simulink model "stereo_ibvs_core_backup_20260724_010158"  (R2025b)
settings: Solver=FixedStepDiscrete  StartTime=0.0  StopTime=10  FixedStep=cfg.Ts  RelTol=1e-3
InitFcn:
  | modelPath = get_param(bdroot,'FileName');
  |                                                                                       simulinkPath = fileparts(fileparts(modelPath));
  |                                                                                       configPath = fullfile(simulinkPath,'config','stereo_ibvs_config.m');
  |                                                                                       if ~isfile(configPath), error('StereoIBVS:ConfigNotFound','找不到配置文件：%s',configPath); end
  |                                                                                       run(configPath);
undefined symbols (not defined in the file): cfg
(part 3 of 4)

== matlab function stereo_ibvs_core_backup_20260724_010158/08_Zoom_Controller/08A Right Visibility Guard/Right Visibility Guard ==
  data: xLeftMeasured input; uRightPredicted output; rhoHatSafe input; focalLengthMeasuredMm input; focalLengthDataValid input; cameraModelValid input; validLeft input; validRight input; ekfPredictionValid input; rightReacquireActive input; resetSafe input; scaleDesired input; numericalEpsilon input; baseline input; outputPixelPitchXmm input; cxR input; focalLengthHardwareMaxMm input; visibilityEpsilon input; imageWidthPx input; rightVisibilityMarginPx input; focalLengthWorkingMaxMm input; focalLengthWorkingMinMm input; targetCharacteristicSize input; rightVisibilityHysteresisPx input; rightVisibilityMarginActualPx output; fRightMaxVisibleMm output; fRightMaxEffectiveMm output; rightScaleDesiredEffective output; rightVisibilityActive output; rightVisibilityInfeasible output; scaleDesiredEffective output; rightScaleDesiredNominal output; fRightMeasuredMm output
function [ ...
    uRightPredicted, ...
    rightVisibilityMarginActualPx, ...
    fRightMaxVisibleMm, ...
    fRightMaxEffectiveMm, ...
    rightScaleDesiredEffective, ...
    rightVisibilityActive, ...
    rightVisibilityInfeasible, ...
    scaleDesiredEffective, ...
    rightScaleDesiredNominal, ...
    fRightMeasuredMm] = fcn( ...
    xLeftMeasured, ...
    rhoHatSafe, ...
    focalLengthMeasuredMm, ...
    focalLengthDataValid, ...
    cameraModelValid, ...
    validLeft, ...
    validRight, ...
    ekfPredictionValid, ...
    rightReacquireActive, ...
    resetSafe, ...
    scaleDesired, ...
    numericalEpsilon, ...
    baseline, ...
    outputPixelPitchXmm, ...
    cxR, ...
    focalLengthHardwareMaxMm, ...
    visibilityEpsilon, ...
    imageWidthPx, ...
    rightVisibilityMarginPx, ...
    focalLengthWorkingMaxMm, ...
    focalLengthWorkingMinMm, ...
    targetCharacteristicSize, ...
    rightVisibilityHysteresisPx)
%#codegen
% 右相机可见性保护。
% 所有配置参数均由外部 Constant 块输入。

persistent active

if isempty(active)
    active = 1;
end

if resetSafe > 0.5
    active = 1;
end

%% 默认安全输出
uRightPredicted = cxR;
rightVisibilityMarginActualPx = 0;

fRightMaxVisibleMm = 0;
fRightMaxEffectiveMm = ...
    focalLengthWorkingMinMm(2);

rightScaleDesiredNominal = ...
    scaleDesired(2);

rightScaleDesiredEffective = ...
    rightScaleDesiredNominal;

scaleDesiredEffective = ...
    scaleDesired;

rightVisibilityActive = 1;
rightVisibilityInfeasible = 1;

fRightMeasuredMm = 0;

%% 输入检查
inputFinite = ...
    isfinite(xLeftMeasured) && ...
    isfinite(rhoHatSafe) && ...
    all(isfinite(focalLengthMeasuredMm)) && ...
    all(isfinite(scaleDesired)) && ...
    isfinite(numericalEpsilon) && ...
    isfinite(baseline) && ...
    isfinite(outputPixelPitchXmm) && ...
    isfinite(cxR) && ...
    all(isfinite(focalLengthHardwareMaxMm)) && ...
    isfinite(visibilityEpsilon) && ...
    isfinite(imageWidthPx) && ...
    isfinite(rightVisibilityMarginPx) && ...
    all(isfinite(focalLengthWorkingMaxMm)) && ...
    all(isfinite(focalLengthWorkingMinMm)) && ...
    isfinite(targetCharacteristicSize) && ...
    isfinite(rightVisibilityHysteresisPx);

modelReady = ...
    focalLengthDataValid > 0.5 && ...
    cameraModelValid > 0.5 && ...
    outputPixelPitchXmm > numericalEpsilon;

if ~inputFinite || ~modelReady
    active = 1;
    return;
end

%% 右相机预测位置
fRightMeasuredMm = ...
    focalLengthMeasuredMm(2);

rho = max( ...
    rhoHatSafe, ...
    numericalEpsilon);

xRightPredicted = ...
    xLeftMeasured - ...
    baseline * rho;

fRightPx = ...
    focalLengthMeasuredMm(2) / ...
    outputPixelPitchXmm;

uRightPredicted = ...
    cxR + ...
    fRightPx * xRightPredicted;

rightVisibilityMarginActualPx = min( ...
    uRightPredicted, ...
    imageWidthPx - uRightPredicted);

%% 可见焦距上限
hardwareMaxPx = ...
    focalLengthHardwareMaxMm(2) / ...
    outputPixelPitchXmm;

if xRightPredicted < -visibilityEpsilon

    fMaxPx = ...
        (cxR - rightVisibilityMarginPx) / ...
        (-xRightPredicted);

elseif xRightPredicted > visibilityEpsilon

    fMaxPx = ...
        (imageWidthPx - ...
        rightVisibilityMarginPx - ...
        cxR) / ...
        xRightPredicted;

else
    fMaxPx = hardwareMaxPx;
end

fMaxPx = max(fMaxPx, 0);

fRightMaxVisibleMm = ...
    fMaxPx * outputPixelPitchXmm;

rawEffectiveMaxMm = min([
    focalLengthWorkingMaxMm(2)
    focalLengthHardwareMaxMm(2)
    fRightMaxVisibleMm
]);

rightVisibilityInfeasible = double( ...
    rawEffectiveMaxMm < ...
    focalLengthWorkingMinMm(2));

fRightMaxEffectiveMm = max( ...
    focalLengthWorkingMinMm(2), ...
    rawEffectiveMaxMm);

%% 调整右相机期望尺度
scaleRightMaxVisible = ...
    targetCharacteristicSize * ...
    fMaxPx * rho;

rightScaleDesiredEffective = min( ...
    rightScaleDesiredNominal, ...
    max(scaleRightMaxVisible, numericalEpsilon));

scaleDesiredEffective = [
    scaleDesired(1)
    rightScaleDesiredEffective
];

%% 滞回状态
enterGuard = ...
    validLeft <= 0.5 || ...
    validRight <= 0.5 || ...
    ekfPredictionValid <= 0.5 || ...
    rightReacquireActive > 0.5 || ...
    rightVisibilityInfeasible > 0.5 || ...
    uRightPredicted < rightVisibilityMarginPx || ...
    uRightPredicted > ...
        imageWidthPx - rightVisibilityMarginPx || ...
    focalLengthMeasuredMm(2) > ...
        fRightMaxEffectiveMm + numericalEpsilon;

exitGuard = ...
    validLeft > 0.5 && ...
    validRight > 0.5 && ...
    ekfPredictionValid > 0.5 && ...
    rightReacquireActive <= 0.5 && ...
    rightVisibilityInfeasible <= 0.5 && ...
    uRightPredicted >= ...
        rightVisibilityMarginPx + ...
        rightVisibilityHysteresisPx && ...
    uRightPredicted <= ...
        imageWidthPx - ...
        rightVisibilityMarginPx - ...
        rightVisibilityHysteresisPx && ...
    focalLengthMeasuredMm(2) <= ...
        fRightMaxEffectiveMm;

if enterGuard
    active = 1;
elseif exitGuard
    active = 0;
end

rightVisibilityActive = ...
    double(active > 0.5);

%% 输出保护
if any(~isfinite([
        uRightPredicted
        rightVisibilityMarginActualPx
        fRightMaxVisibleMm
        fRightMaxEffectiveMm
        rightScaleDesiredEffective
        scaleDesiredEffective
        fRightMeasuredMm]))

    active = 1;

    uRightPredicted = cxR;
    rightVisibilityMarginActualPx = 0;

    fRightMaxVisibleMm = 0;
    fRightMaxEffectiveMm = ...
        focalLengthWorkingMinMm(2);

    rightScaleDesiredEffective = ...
        numericalEpsilon;

    scaleDesiredEffective = [
        scaleDesired(1)
        rightScaleDesiredEffective
    ];

    rightVisibilityActive = 1;
    rightVisibilityInfeasible = 1;
    fRightMeasuredMm = 0;
end
end

== matlab function stereo_ibvs_core_backup_20260724_010158/08_Zoom_Controller/08B_Zoom_Controller_Mm/V2 Zoom Controller ==
  data: focalLengthMeasuredMm input; fDotMmCmd output; focalLengthFresh input; focalLengthDataValid input; cameraModelValid input; scaleMeasured input; rhoHatSafe input; rhoDotHat input; scaleDesiredEffective input; validLeft input; ekfPredictionValid input; focalAtWorkingLowerLimit input; focalAtWorkingUpperLimit input; fRightMaxEffectiveMm input; rightVisibilityActive input; rightReacquireActive input; numericalEpsilon input; focalLengthWorkingMaxMm input; robustEnable input; betaF input; epsilonF input; Kf input; targetCharacteristicSize input; outputPixelPitchXmm input; focalLengthWorkingMinMm input; rightReacquireZoomRateMmPerSec input; focalRateDesignMmPerSec input; Ts input; focalRateGuaranteedMmPerSec input; focalRateAbsoluteMaxMmPerSec input; zoomControlEnable input; fDotMmLimited output; scaleError output; gDotCmd output; focalCommandOutwardAtWorkingLimit output; focalFeasible output; focalRateUsageGuaranteedCmd output; focalRateUsageHardCmd output
function [ ...
    fDotMmCmd, ...
    fDotMmLimited, ...
    scaleError, ...
    gDotCmd, ...
    focalCommandOutwardAtWorkingLimit, ...
    focalFeasible, ...
    focalRateUsageGuaranteedCmd, ...
    focalRateUsageHardCmd] = fcn( ...
    focalLengthMeasuredMm, ...
    focalLengthFresh, ...
    focalLengthDataValid, ...
    cameraModelValid, ...
    scaleMeasured, ...
    rhoHatSafe, ...
    rhoDotHat, ...
    scaleDesiredEffective, ...
    validLeft, ...
    ekfPredictionValid, ...
    focalAtWorkingLowerLimit, ...
    focalAtWorkingUpperLimit, ...
    fRightMaxEffectiveMm, ...
    rightVisibilityActive, ...
    rightReacquireActive, ...
    numericalEpsilon, ...
    focalLengthWorkingMaxMm, ...
    robustEnable, ...
    betaF, ...
    epsilonF, ...
    Kf, ...
    targetCharacteristicSize, ...
    outputPixelPitchXmm, ...
    focalLengthWorkingMinMm, ...
    rightReacquireZoomRateMmPerSec, ...
    focalRateDesignMmPerSec, ...
    Ts, ...
    focalRateGuaranteedMmPerSec, ...
    focalRateAbsoluteMaxMmPerSec, ...
    zoomControlEnable)
%#codegen
% V2 Zoom控制器。
% 焦距单位mm，速度命令单位mm/s。
% 所有配置参数均由外部 Constant 块输入。

%% 固定尺寸输出
fDotMmCmd = zeros(2,1);
fDotMmLimited = zeros(2,1);

scaleError = zeros(2,1);
gDotCmd = zeros(2,1);

focalCommandOutwardAtWorkingLimit = ...
    zeros(2,1);

focalFeasible = zeros(2,1);

focalRateUsageGuaranteedCmd = ...
    zeros(2,1);

focalRateUsageHardCmd = ...
    zeros(2,1);

%% 输入检查
inputFinite = ...
    all(isfinite(focalLengthMeasuredMm)) && ...
    all(isfinite(scaleMeasured)) && ...
    isfinite(rhoHatSafe) && ...
    all(isfinite(rhoDotHat)) && ...
    all(isfinite(scaleDesiredEffective)) && ...
    all(isfinite(focalAtWorkingLowerLimit)) && ...
    all(isfinite(focalAtWorkingUpperLimit)) && ...
    isfinite(fRightMaxEffectiveMm) && ...
    isfinite(numericalEpsilon) && ...
    all(isfinite(focalLengthWorkingMaxMm)) && ...
    isfinite(robustEnable) && ...
    all(isfinite(betaF)) && ...
    all(isfinite(epsilonF)) && ...
    all(isfinite(Kf(:))) && ...
    isfinite(targetCharacteristicSize) && ...
    isfinite(outputPixelPitchXmm) && ...
    all(isfinite(focalLengthWorkingMinMm)) && ...
    isfinite(rightReacquireZoomRateMmPerSec) && ...
    isfinite(focalRateDesignMmPerSec) && ...
    isfinite(Ts) && ...
    isfinite(focalRateGuaranteedMmPerSec) && ...
    isfinite(focalRateAbsoluteMaxMmPerSec) && ...
    isfinite(zoomControlEnable);

if ~inputFinite || ...
        numericalEpsilon <= 0 || ...
        outputPixelPitchXmm <= numericalEpsilon || ...
        Ts <= 0

    return;
end

rho = max(rhoHatSafe, numericalEpsilon);

upperEffectiveMm = [
    focalLengthWorkingMaxMm(1)
    fRightMaxEffectiveMm
];

%% V2控制律
for cameraIndex = 1:2

    scaleCurrent = max( ...
        scaleMeasured(cameraIndex), ...
        numericalEpsilon);

    scaleDesiredCurrent = max( ...
        scaleDesiredEffective(cameraIndex), ...
        numericalEpsilon);

    scaleError(cameraIndex) = ...
        log(scaleCurrent / scaleDesiredCurrent);

    depthRateEstimate = ...
        rhoDotHat(cameraIndex) / rho;

    robustTerm = 0;

    if robustEnable > 0.5
        robustTerm = ...
            betaF(cameraIndex) * ...
            scaleError(cameraIndex) / ...
            (abs(scaleError(cameraIndex)) + ...
            epsilonF(cameraIndex));
    end

    gDotCmd(cameraIndex) = ...
        -Kf(cameraIndex,cameraIndex) * ...
        scaleError(cameraIndex) - ...
        depthRateEstimate - ...
        robustTerm;

    fDotMmCmd(cameraIndex) = ...
        focalLengthMeasuredMm(cameraIndex) * ...
        gDotCmd(cameraIndex);

    focalRequiredMm = ...
        scaleDesiredEffective(cameraIndex) / ...
        (targetCharacteristicSize * rho) * ...
        outputPixelPitchXmm;

    focalFeasible(cameraIndex) = double( ...
        focalRequiredMm >= ...
            focalLengthWorkingMinMm(cameraIndex) && ...
        focalRequiredMm <= ...
            upperEffectiveMm(cameraIndex));
end

%% 焦距反馈超时或模型失效：Zoom立即停止
zoomInputValid = ...
    focalLengthFresh > 0.5 && ...
    focalLengthDataValid > 0.5 && ...
    cameraModelValid > 0.5;

if ~zoomInputValid || ...
        zoomControlEnable <= 0.5

    fDotMmCmd = zeros(2,1);
    fDotMmLimited = zeros(2,1);
    gDotCmd = zeros(2,1);
    return;
end

%% 右相机可见性保护
if rightVisibilityActive > 0.5 || ...
        rightReacquireActive > 0.5

    if focalLengthMeasuredMm(2) > ...
            fRightMaxEffectiveMm + numericalEpsilon

        fDotMmCmd(2) = ...
            -rightReacquireZoomRateMmPerSec;
    else
        fDotMmCmd(2) = ...
            min(fDotMmCmd(2), 0);
    end
end

%% 左相机或EKF无效：保留V2安全缩焦
if validLeft <= 0.5 || ...
        ekfPredictionValid <= 0.5

    fDotMmCmd = zeros(2,1);

    for cameraIndex = 1:2
        if focalLengthMeasuredMm(cameraIndex) > ...
                focalLengthWorkingMinMm(cameraIndex)

            fDotMmCmd(cameraIndex) = ...
                -rightReacquireZoomRateMmPerSec;
        end
    end
end

%% 工作范围方向诊断
for cameraIndex = 1:2

    focalCommandOutwardAtWorkingLimit(cameraIndex) = ...
        double( ...
        (focalAtWorkingLowerLimit(cameraIndex) > 0.5 && ...
        fDotMmCmd(cameraIndex) < 0) || ...
        (focalAtWorkingUpperLimit(cameraIndex) > 0.5 && ...
        fDotMmCmd(cameraIndex) > 0) || ...
        (focalLengthMeasuredMm(cameraIndex) >= ...
        upperEffectiveMm(cameraIndex) && ...
        fDotMmCmd(cameraIndex) > 0));
end

%% V2设计速度限制
fDotMmLimited = min( ...
    max( ...
        fDotMmCmd, ...
        -focalRateDesignMmPerSec), ...
    focalRateDesignMmPerSec);

%% 防止下一周期越过右相机可见焦距上限
nextRightFocalLengthMm = ...
    focalLengthMeasuredMm(2) + ...
    Ts * fDotMmLimited(2);

if focalLengthMeasuredMm(2) <= ...
        fRightMaxEffectiveMm && ...
        nextRightFocalLengthMm > ...
        fRightMaxEffectiveMm

    fDotMmLimited(2) = min( ...
        fDotMmLimited(2), ...
        (fRightMaxEffectiveMm - ...
        focalLengthMeasuredMm(2)) / Ts);
end

%% 速度使用率
if focalRateGuaranteedMmPerSec > numericalEpsilon
    focalRateUsageGuaranteedCmd = ...
        abs(fDotMmLimited) / ...
        focalRateGuaranteedMmPerSec;
end

if focalRateAbsoluteMaxMmPerSec > numericalEpsilon
    focalRateUsageHardCmd = ...
        abs(fDotMmLimited) / ...
        focalRateAbsoluteMaxMmPerSec;
end

%% 输出有限值保护
if any(~isfinite(fDotMmCmd)) || ...
        any(~isfinite(fDotMmLimited)) || ...
        any(~isfinite(scaleError)) || ...
        any(~isfinite(gDotCmd)) || ...
        any(~isfinite(focalFeasible)) || ...
        any(~isfinite(focalRateUsageGuaranteedCmd)) || ...
        any(~isfinite(focalRateUsageHardCmd))

    fDotMmCmd = zeros(2,1);
    fDotMmLimited = zeros(2,1);

    scaleError = zeros(2,1);
    gDotCmd = zeros(2,1);

    focalCommandOutwardAtWorkingLimit = ...
        zeros(2,1);

    focalFeasible = zeros(2,1);

    focalRateUsageGuaranteedCmd = ...
        zeros(2,1);

    focalRateUsageHardCmd = ...
        zeros(2,1);
end
end

== matlab function stereo_ibvs_core_backup_20260724_010158/08_Zoom_Controller/08C_Zoom_Priority_Supervisor/V2 Zoom Priority Supervisor ==
  data: scaleError input; depthTaskWeight output; depthErrorDelayed input; focalLengthMeasuredMm input; focalLengthFresh input; focalLengthDataValid input; cameraModelValid input; focalAtWorkingLowerLimit input; focalAtWorkingUpperLimit input; focalHeadroomMm input; focalFeasible input; validLeft input; validStereoQualified input; ekfPredictionValid input; resetSafe input; focalCommandOutwardAtWorkingLimit input; focalRateUsageGuaranteedCmd input; focalRateUsageHardCmd input; rightReacquireActive input; Ts input; zoomPriorityEnable input; armDepthRampTime input; scaleErrorEnterThreshold input; scaleErrorExitThreshold input; scaleSettledHoldTime input; disturbanceConfirmTime input; zoomOnlyMaxTime input; schedulerMode output; zoomPriorityActive output; zoomPriorityTimer output; scaleSettledTimer output; armRecoveryReason output; newDisturbanceDetected output
function [ ...
    depthTaskWeight, ...
    schedulerMode, ...
    zoomPriorityActive, ...
    zoomPriorityTimer, ...
    scaleSettledTimer, ...
    armRecoveryReason, ...
    newDisturbanceDetected] = fcn( ...
    scaleError, ...
    depthErrorDelayed, ...
    focalLengthMeasuredMm, ...
    focalLengthFresh, ...
    focalLengthDataValid, ...
    cameraModelValid, ...
    focalAtWorkingLowerLimit, ...
    focalAtWorkingUpperLimit, ...
    focalHeadroomMm, ...
    focalFeasible, ...
    validLeft, ...
    validStereoQualified, ...
    ekfPredictionValid, ...
    resetSafe, ...
    focalCommandOutwardAtWorkingLimit, ...
    focalRateUsageGuaranteedCmd, ...
    focalRateUsageHardCmd, ...
    rightReacquireActive, ...
    Ts, ...
    zoomPriorityEnable, ...
    armDepthRampTime, ...
    scaleErrorEnterThreshold, ...
    scaleErrorExitThreshold, ...
    scaleSettledHoldTime, ...
    disturbanceConfirmTime, ...
    zoomOnlyMaxTime)
%#codegen
% V2 Zoom优先级状态机。
% 所有配置参数均由外部 Constant 块输入。
%
% schedulerMode:
% 0 INITIALIZE
% 1 ZOOM_FIRST
% 2 ARM_RECOVERY
% 3 FULL_TRACK
% 4 SAFE_HOLD
% 5 RIGHT_REACQUIRE

persistent mode
persistent zoomTimer
persistent settledTimer
persistent rampTimer
persistent reason
persistent disturbanceTimer
persistent validLast
persistent rateTimer

if isempty(mode)
    mode = 0;
    zoomTimer = 0;
    settledTimer = 0;
    rampTimer = 0;
    reason = 0;
    disturbanceTimer = 0;
    validLast = 0;
    rateTimer = 0;
end

if resetSafe > 0.5
    mode = 0;
    zoomTimer = 0;
    settledTimer = 0;
    rampTimer = 0;
    reason = 0;
    disturbanceTimer = 0;
    validLast = 0;
    rateTimer = 0;
end

depthTaskWeight = 0;
newDisturbanceDetected = 0;

centerValid = ...
    validLeft > 0.5;

focalStateValid = ...
    focalLengthDataValid > 0.5 && ...
    cameraModelValid > 0.5;

depthReady = ...
    validStereoQualified > 0.5 && ...
    ekfPredictionValid > 0.5 && ...
    rightReacquireActive <= 0.5;

maximumScaleError = ...
    max(abs(scaleError));

%% 中心任务无效
if ~centerValid

    mode = 4;
    depthTaskWeight = 0;

    zoomTimer = 0;
    settledTimer = 0;
    rampTimer = 0;
    disturbanceTimer = 0;
    rateTimer = 0;
    validLast = 0;

%% 焦距数据或相机模型无效
elseif ~focalStateValid

    mode = 4;
    depthTaskWeight = 0;

    zoomTimer = 0;
    settledTimer = 0;
    rampTimer = 0;
    disturbanceTimer = 0;
    rateTimer = 0;
    validLast = 0;

%% 双目深度暂不可用
elseif ~depthReady

    mode = 5;
    depthTaskWeight = 0;

    zoomTimer = 0;
    settledTimer = 0;
    rampTimer = 0;
    disturbanceTimer = 0;
    rateTimer = 0;
    validLast = 0;

%% 焦距仅不新鲜：Zoom暂停，深度继续
elseif focalLengthFresh <= 0.5

    mode = 3;
    depthTaskWeight = 1;

    zoomTimer = 0;
    settledTimer = 0;
    rampTimer = armDepthRampTime;
    disturbanceTimer = 0;
    rateTimer = 0;
    reason = 0;
    validLast = 1;

%% 禁用Zoom优先级
elseif zoomPriorityEnable <= 0.5

    mode = 3;
    depthTaskWeight = 1;

    zoomTimer = 0;
    settledTimer = 0;
    rampTimer = armDepthRampTime;
    disturbanceTimer = 0;
    rateTimer = 0;
    reason = 0;
    validLast = 1;

else

    if validLast < 0.5 && ...
            (mode == 4 || mode == 5)

        mode = 1;

        zoomTimer = 0;
        settledTimer = 0;
        rampTimer = 0;
        disturbanceTimer = 0;
        rateTimer = 0;
        reason = 0;
    end

    if mode == 0

        if maximumScaleError > ...
                scaleErrorEnterThreshold

            mode = 1;
            depthTaskWeight = 0;

        else
            mode = 3;
            depthTaskWeight = 1;
        end

    elseif mode == 1

        depthTaskWeight = 0;
        zoomTimer = zoomTimer + Ts;

        if maximumScaleError <= ...
                scaleErrorExitThreshold

            settledTimer = ...
                settledTimer + Ts;
        else
            settledTimer = 0;
        end

        if any( ...
                focalRateUsageGuaranteedCmd >= 1)

            rateTimer = ...
                rateTimer + Ts;
        else
            rateTimer = 0;
        end

        if any(focalRateUsageHardCmd >= 1)

            mode = 2;
            reason = 6;
            rampTimer = 0;
            rateTimer = 0;

        elseif rateTimer >= ...
                disturbanceConfirmTime && ...
                maximumScaleError > ...
                scaleErrorExitThreshold

            mode = 2;
            reason = 5;
            rampTimer = 0;
            rateTimer = 0;

        elseif settledTimer >= ...
                scaleSettledHoldTime

            mode = 2;
            reason = 1;
            rampTimer = 0;
            rateTimer = 0;

        elseif any( ...
                focalCommandOutwardAtWorkingLimit > 0.5)

            mode = 2;
            reason = 7;
            rampTimer = 0;
            rateTimer = 0;

        elseif zoomTimer >= ...
                disturbanceConfirmTime && ...
                any(focalFeasible < 0.5)

            mode = 2;
            reason = 3;
            rampTimer = 0;
            rateTimer = 0;

        elseif zoomTimer >= zoomOnlyMaxTime

            mode = 2;
            reason = 4;
            rampTimer = 0;
            rateTimer = 0;
        end

    elseif mode == 2

        rampTimer = min( ...
            rampTimer + Ts, ...
            armDepthRampTime);

        rampFraction = min(max( ...
            rampTimer / max( ...
                armDepthRampTime, ...
                Ts), ...
            0), 1);

        depthTaskWeight = ...
            rampFraction * ...
            rampFraction * ...
            (3 - 2*rampFraction);

        if depthTaskWeight >= 1 - 1e-6
            mode = 3;
            depthTaskWeight = 1;
            disturbanceTimer = 0;
        end

    elseif mode == 3

        depthTaskWeight = 1;

        if maximumScaleError >= ...
                scaleErrorEnterThreshold

            depthTaskWeight = 0;

            disturbanceTimer = ...
                disturbanceTimer + Ts;
        else
            disturbanceTimer = 0;
        end

        if disturbanceTimer >= ...
                disturbanceConfirmTime

            mode = 1;
            depthTaskWeight = 0;

            zoomTimer = 0;
            settledTimer = 0;
            rampTimer = 0;
            disturbanceTimer = 0;
            rateTimer = 0;
            reason = 0;

            newDisturbanceDetected = 1;
        end

    else

        mode = 1;
        depthTaskWeight = 0;

        zoomTimer = 0;
        settledTimer = 0;
        rampTimer = 0;
        disturbanceTimer = 0;
        rateTimer = 0;
        reason = 0;
    end

    validLast = 1;
end

schedulerMode = mode;

zoomPriorityActive = ...
    double(mode == 1);

zoomPriorityTimer = ...
    zoomTimer;

scaleSettledTimer = ...
    settledTimer;

armRecoveryReason = ...
    reason;

%% 有限值保护
diagnosticFinite = all(isfinite([
    depthTaskWeight
    schedulerMode
    zoomPriorityTimer
    scaleSettledTimer
    depthErrorDelayed
    focalLengthMeasuredMm
    focalHeadroomMm
    focalAtWorkingLowerLimit
    focalAtWorkingUpperLimit
    focalLengthFresh
    focalLengthDataValid
    cameraModelValid
    Ts
    zoomPriorityEnable
    armDepthRampTime
    scaleErrorEnterThreshold
    scaleErrorExitThreshold
    scaleSettledHoldTime
    disturbanceConfirmTime
    zoomOnlyMaxTime
]));

if ~diagnosticFinite

    mode = 4;
    zoomTimer = 0;
    settledTimer = 0;
    rampTimer = 0;
    reason = 0;
    disturbanceTimer = 0;
    validLast = 0;
    rateTimer = 0;

    depthTaskWeight = 0;
    schedulerMode = 4;
    zoomPriorityActive = 0;
    zoomPriorityTimer = 0;
    scaleSettledTimer = 0;
    armRecoveryReason = 0;
    newDisturbanceDetected = 0;
end
end

== matlab function stereo_ibvs_core_backup_20260724_010158/09_Safety_Supervisor/Apply Safety and Saturation ==
  data: qDotCmd input; qDotApplied output; fDotMmLimited input; q input; focalLengthMeasuredMm input; validLeft input; focalLengthFresh input; cameraModelValid input; kinematicsValid input; JL input; controllerEnableSafe input; cfg_qDotMax input; cfg_qDotAlgorithmMax input; cfg_qMin input; cfg_qMax input; cfg_qLimitSoftMargin input; cfg_cartesianLinearSpeedMax input; cfg_focalRateGuaranteedMmPerSec input; cfg_focalRateAbsoluteMaxMmPerSec input; cfg_focalLengthWorkingMinMm input; cfg_focalLengthWorkingMaxMm input; cfg_focalLengthHardwareMinMm input; cfg_focalLengthHardwareMaxMm input; cfg_Ts input; cfg_numericalEpsilon input; cfg_armControlCalibrationReady input; cfg_zoomControlCalibrationReady input; cfg_armControlEnable input; cfg_zoomControlEnable input; fDotMmApplied output; qSaturationFlag output; focalRateSaturationFlag output; jointVelocitySaturationFlag output; jointVelocitySaturationAny output; jointLimitWarning output; cartesianSpeed output; cartesianSpeedScale output; cartesianSpeedSaturationFlag output; focalLengthCommandMm output; focalRateUsageGuaranteed output; focalRateUsageHard output; focalRateHardViolation output; safetyValid output
function [ ...
    qDotApplied, ...
    fDotMmApplied, ...
    qSaturationFlag, ...
    focalRateSaturationFlag, ...
    jointVelocitySaturationFlag, ...
    jointVelocitySaturationAny, ...
    jointLimitWarning, ...
    cartesianSpeed, ...
    cartesianSpeedScale, ...
    cartesianSpeedSaturationFlag, ...
    focalLengthCommandMm, ...
    focalRateUsageGuaranteed, ...
    focalRateUsageHard, ...
    focalRateHardViolation, ...
    safetyValid] = fcn( ...
    qDotCmd, ...
    fDotMmLimited, ...
    q, ...
    focalLengthMeasuredMm, ...
    validLeft, ...
    focalLengthFresh, ...
    cameraModelValid, ...
    kinematicsValid, ...
    JL, ...
    controllerEnableSafe, ...
    cfg_qDotMax, ...
    cfg_qDotAlgorithmMax, ...
    cfg_qMin, ...
    cfg_qMax, ...
    cfg_qLimitSoftMargin, ...
    cfg_cartesianLinearSpeedMax, ...
    cfg_focalRateGuaranteedMmPerSec, ...
    cfg_focalRateAbsoluteMaxMmPerSec, ...
    cfg_focalLengthWorkingMinMm, ...
    cfg_focalLengthWorkingMaxMm, ...
    cfg_focalLengthHardwareMinMm, ...
    cfg_focalLengthHardwareMaxMm, ...
    cfg_Ts, ...
    cfg_numericalEpsilon, ...
    cfg_armControlCalibrationReady, ...
    cfg_zoomControlCalibrationReady, ...
    cfg_armControlEnable, ...
    cfg_zoomControlEnable)
%#codegen
% V2 Safety and Saturation
% JL顺序：[linear velocity; angular velocity]

%% 固定尺寸输出
qDotApplied = zeros(7,1);
fDotMmApplied = zeros(2,1);

qSaturationFlag = 0;
focalRateSaturationFlag = 0;

jointVelocitySaturationFlag = zeros(7,1);
jointVelocitySaturationAny = 0;
jointLimitWarning = zeros(7,1);

cartesianSpeed = 0;
cartesianSpeedScale = 1;
cartesianSpeedSaturationFlag = 0;

focalLengthCommandMm = zeros(2,1);
focalRateUsageGuaranteed = zeros(2,1);
focalRateUsageHard = zeros(2,1);
focalRateHardViolation = zeros(2,1);

safetyValid = 0;

%% 固定尺寸输入
qDotRequested = reshape(qDotCmd,7,1);
fDotRequested = reshape(fDotMmLimited,2,1);
qMeasured = reshape(q,7,1);
focalMeasured = reshape(focalLengthMeasuredMm,2,1);

%% 参数检查
tol = max(cfg_numericalEpsilon,1e-12);

inputFinite = ...
    all(isfinite(qDotRequested)) && ...
    all(isfinite(fDotRequested)) && ...
    all(isfinite(qMeasured)) && ...
    all(isfinite(focalMeasured)) && ...
    all(isfinite(JL(:))) && ...
    isfinite(validLeft) && ...
    isfinite(focalLengthFresh) && ...
    isfinite(cameraModelValid) && ...
    isfinite(kinematicsValid) && ...
    isfinite(controllerEnableSafe);

parameterFinite = ...
    all(isfinite(cfg_qDotMax)) && ...
    all(isfinite(cfg_qDotAlgorithmMax)) && ...
    all(isfinite(cfg_qMin)) && ...
    all(isfinite(cfg_qMax)) && ...
    isfinite(cfg_qLimitSoftMargin) && ...
    isfinite(cfg_cartesianLinearSpeedMax) && ...
    isfinite(cfg_focalRateGuaranteedMmPerSec) && ...
    isfinite(cfg_focalRateAbsoluteMaxMmPerSec) && ...
    all(isfinite(cfg_focalLengthWorkingMinMm)) && ...
    all(isfinite(cfg_focalLengthWorkingMaxMm)) && ...
    all(isfinite(cfg_focalLengthHardwareMinMm)) && ...
    all(isfinite(cfg_focalLengthHardwareMaxMm)) && ...
    isfinite(cfg_Ts) && ...
    isfinite(cfg_numericalEpsilon) && ...
    isfinite(cfg_armControlCalibrationReady) && ...
    isfinite(cfg_zoomControlCalibrationReady) && ...
    isfinite(cfg_armControlEnable) && ...
    isfinite(cfg_zoomControlEnable);

parameterRangesValid = ...
    all(cfg_qDotMax >= 0) && ...
    all(cfg_qDotAlgorithmMax >= 0) && ...
    all(cfg_qMax > cfg_qMin) && ...
    cfg_qLimitSoftMargin >= 0 && ...
    all(2*cfg_qLimitSoftMargin < ...
        (cfg_qMax-cfg_qMin)) && ...
    cfg_cartesianLinearSpeedMax > 0 && ...
    cfg_focalRateGuaranteedMmPerSec > 0 && ...
    cfg_focalRateAbsoluteMaxMmPerSec >= ...
        cfg_focalRateGuaranteedMmPerSec && ...
    all(cfg_focalLengthHardwareMaxMm > ...
        cfg_focalLengthHardwareMinMm) && ...
    all(cfg_focalLengthWorkingMinMm >= ...
        cfg_focalLengthHardwareMinMm) && ...
    all(cfg_focalLengthWorkingMaxMm <= ...
        cfg_focalLengthHardwareMaxMm) && ...
    all(cfg_focalLengthWorkingMaxMm > ...
        cfg_focalLengthWorkingMinMm) && ...
    cfg_Ts > 0;

if ~(inputFinite && parameterFinite && parameterRangesValid)
    qSaturationFlag = 1;
    focalRateSaturationFlag = 1;
    jointVelocitySaturationFlag = ones(7,1);
    jointVelocitySaturationAny = 1;
    cartesianSpeedScale = 0;
    return;
end

safetyValid = 1;

%% 当前焦距
if cameraModelValid > 0.5
    focalLengthCommandMm = focalMeasured;
end

%% 关节限位诊断
for i = 1:7
    nearLowerLimit = ...
        qMeasured(i) <= ...
        cfg_qMin(i)+cfg_qLimitSoftMargin;

    nearUpperLimit = ...
        qMeasured(i) >= ...
        cfg_qMax(i)-cfg_qLimitSoftMargin;

    outsideLowerLimit = ...
        qMeasured(i) <= cfg_qMin(i);

    outsideUpperLimit = ...
        qMeasured(i) >= cfg_qMax(i);

    jointLimitWarning(i) = double( ...
        nearLowerLimit || ...
        nearUpperLimit || ...
        outsideLowerLimit || ...
        outsideUpperLimit);
end

%% 控制许可
armPermission = ...
    controllerEnableSafe > 0.5 && ...
    cfg_armControlEnable > 0.5 && ...
    cfg_armControlCalibrationReady > 0.5 && ...
    validLeft > 0.5 && ...
    cameraModelValid > 0.5 && ...
    kinematicsValid > 0.5;

zoomPermission = ...
    controllerEnableSafe > 0.5 && ...
    cfg_zoomControlEnable > 0.5 && ...
    cfg_zoomControlCalibrationReady > 0.5 && ...
    validLeft > 0.5 && ...
    cameraModelValid > 0.5 && ...
    focalLengthFresh > 0.5;

%% 关节速度限制
if armPermission

    qDotLimit = min( ...
        abs(cfg_qDotMax), ...
        abs(cfg_qDotAlgorithmMax));

    qCandidate = min( ...
        max(qDotRequested,-qDotLimit), ...
        qDotLimit);

    for i = 1:7

        nearLowerLimit = ...
            qMeasured(i) <= ...
            cfg_qMin(i)+cfg_qLimitSoftMargin;

        nearUpperLimit = ...
            qMeasured(i) >= ...
            cfg_qMax(i)-cfg_qLimitSoftMargin;

        if nearLowerLimit && qCandidate(i) < 0
            qCandidate(i) = 0;
        end

        if nearUpperLimit && qCandidate(i) > 0
            qCandidate(i) = 0;
        end
    end

    %% 笛卡尔线速度限制
    cameraTwistCandidate = JL*qCandidate;
    cartesianSpeedCandidate = ...
        norm(cameraTwistCandidate(1:3));

    if ~isfinite(cartesianSpeedCandidate)

        qCandidate = zeros(7,1);
        cartesianSpeedScale = 0;
        cartesianSpeedSaturationFlag = 1;
        safetyValid = 0;

    elseif cartesianSpeedCandidate > ...
            cfg_cartesianLinearSpeedMax

        cartesianSpeedScale = ...
            cfg_cartesianLinearSpeedMax / ...
            max(cartesianSpeedCandidate,tol);

        qCandidate = ...
            cartesianSpeedScale*qCandidate;

        cartesianSpeedSaturationFlag = 1;
    end

    qDotApplied = min( ...
        max(qCandidate,-qDotLimit), ...
        qDotLimit);

    finalCameraTwist = JL*qDotApplied;
    cartesianSpeed = norm(finalCameraTwist(1:3));
end

%% Zoom硬限速违规诊断
focalRateHardViolation = double( ...
    abs(fDotRequested) > ...
    cfg_focalRateAbsoluteMaxMmPerSec);

%% Zoom焦距速度限制
if zoomPermission

    fCandidate = min( ...
        max(fDotRequested, ...
            -cfg_focalRateAbsoluteMaxMmPerSec), ...
        cfg_focalRateAbsoluteMaxMmPerSec);

    for i = 1:2

        focalCurrent = focalMeasured(i);

        workingMin = ...
            cfg_focalLengthWorkingMinMm(i);
        workingMax = ...
            cfg_focalLengthWorkingMaxMm(i);

        hardwareMin = ...
            cfg_focalLengthHardwareMinMm(i);
        hardwareMax = ...
            cfg_focalLengthHardwareMaxMm(i);

        %% 禁止继续远离工作范围
        if focalCurrent <= workingMin && ...
                fCandidate(i) < 0
            fCandidate(i) = 0;
        end

        if focalCurrent >= workingMax && ...
                fCandidate(i) > 0
            fCandidate(i) = 0;
        end

        %% 下一周期工作范围预测
        nextFocalLength = ...
            focalCurrent + ...
            cfg_Ts*fCandidate(i);

        if focalCurrent >= workingMin && ...
                nextFocalLength < workingMin

            fCandidate(i) = ...
                (workingMin-focalCurrent)/cfg_Ts;

        elseif focalCurrent <= workingMax && ...
                nextFocalLength > workingMax

            fCandidate(i) = ...
                (workingMax-focalCurrent)/cfg_Ts;
        end

        %% 硬件范围最终保护
        nextFocalLength = ...
            focalCurrent + ...
            cfg_Ts*fCandidate(i);

        if nextFocalLength < hardwareMin

            fCandidate(i) = ...
                (hardwareMin-focalCurrent)/cfg_Ts;

        elseif nextFocalLength > hardwareMax

            fCandidate(i) = ...
                (hardwareMax-focalCurrent)/cfg_Ts;
        end
    end

    fDotMmApplied = min( ...
        max(fCandidate, ...
            -cfg_focalRateAbsoluteMaxMmPerSec), ...
        cfg_focalRateAbsoluteMaxMmPerSec);
end

%% 最终有限值保护
if any(~isfinite(qDotApplied)) || ...
        ~isfinite(cartesianSpeed) || ...
        ~isfinite(cartesianSpeedScale)

    qDotApplied = zeros(7,1);
    cartesianSpeed = 0;
    cartesianSpeedScale = 0;
    cartesianSpeedSaturationFlag = 1;
    safetyValid = 0;
end

if any(~isfinite(fDotMmApplied))
    fDotMmApplied = zeros(2,1);
    safetyValid = 0;
end

%% 饱和诊断
jointVelocitySaturationFlag = double( ...
    abs(qDotApplied-qDotRequested) > tol);

jointVelocitySaturationAny = double( ...
    any(jointVelocitySaturationFlag > 0.5));

qSaturationFlag = ...
    jointVelocitySaturationAny;

focalRateSaturationFlag = double( ...
    any(abs(fDotMmApplied-fDotRequested) > tol));

%% Zoom使用率
focalRateUsageGuaranteed = ...
    abs(fDotMmApplied) / ...
    cfg_focalRateGuaranteedMmPerSec;

focalRateUsageHard = ...
    abs(fDotMmApplied) / ...
    cfg_focalRateAbsoluteMaxMmPerSec;

%% 下一周期焦距命令
if cameraModelValid > 0.5

    focalLengthCommandMm = min( ...
        max( ...
            focalMeasured + ...
            cfg_Ts*fDotMmApplied, ...
            cfg_focalLengthHardwareMinMm), ...
        cfg_focalLengthHardwareMaxMm);

else
    focalLengthCommandMm = zeros(2,1);
end

%% 最终输出检查
if any(~isfinite(focalLengthCommandMm)) || ...
        any(~isfinite(focalRateUsageGuaranteed)) || ...
        any(~isfinite(focalRateUsageHard))

    fDotMmApplied = zeros(2,1);
    focalLengthCommandMm = zeros(2,1);
    focalRateUsageGuaranteed = zeros(2,1);
    focalRateUsageHard = zeros(2,1);
    safetyValid = 0;
end
end

== matlab function stereo_ibvs_core_backup_20260724_010158/10_Diagnostics/V2_Output_and_Diagnostics ==
  data: qDotApplied input; jointVelocityCmd output; fDotMmApplied input; inputDataValid input; cameraModelValid input; focalLengthFresh input; kinematicsValid input; validLeft input; validRight input; validStereoQualified input; ekfPredictionValid input; ekfMeasurementUpdated input; depthTaskWeight input; schedulerMode input; safetyValid input; controllerEnableSafe input; focalRateCmdMmPerSec output; controllerStatus output
function [ ...
    jointVelocityCmd, ...
    focalRateCmdMmPerSec, ...
    controllerStatus] = fcn( ...
    qDotApplied, ...
    fDotMmApplied, ...
    inputDataValid, ...
    cameraModelValid, ...
    focalLengthFresh, ...
    kinematicsValid, ...
    validLeft, ...
    validRight, ...
    validStereoQualified, ...
    ekfPredictionValid, ...
    ekfMeasurementUpdated, ...
    depthTaskWeight, ...
    schedulerMode, ...
    safetyValid, ...
    controllerEnableSafe)
%#codegen
% V2 Output and Diagnostics
%
% jointVelocityCmd:
% [qDot1; ...; qDot7]，单位 rad/s
%
% focalRateCmdMmPerSec:
% [fDotLeft; fDotRight]，单位 mm/s
%
% 不再进行焦距速度到step/s的转换。

%% 固定尺寸输出
jointVelocityCmd = zeros(7,1);
focalRateCmdMmPerSec = zeros(2,1);
controllerStatus = zeros(13,1);

%% 固定尺寸输入
qDot = reshape(qDotApplied,7,1);
fDotMm = reshape(fDotMmApplied,2,1);

%% 状态信号整理
statusInputDataValid = double( ...
    isfinite(inputDataValid) && ...
    inputDataValid > 0.5);

statusCameraModelValid = double( ...
    isfinite(cameraModelValid) && ...
    cameraModelValid > 0.5);

statusFocalLengthFresh = double( ...
    isfinite(focalLengthFresh) && ...
    focalLengthFresh > 0.5);

statusKinematicsValid = double( ...
    isfinite(kinematicsValid) && ...
    kinematicsValid > 0.5);

statusValidLeft = double( ...
    isfinite(validLeft) && ...
    validLeft > 0.5);

statusValidRight = double( ...
    isfinite(validRight) && ...
    validRight > 0.5);

statusValidStereoQualified = double( ...
    isfinite(validStereoQualified) && ...
    validStereoQualified > 0.5);

statusEkfPredictionValid = double( ...
    isfinite(ekfPredictionValid) && ...
    ekfPredictionValid > 0.5);

statusEkfMeasurementUpdated = double( ...
    isfinite(ekfMeasurementUpdated) && ...
    ekfMeasurementUpdated > 0.5);

if isfinite(depthTaskWeight)
    statusDepthTaskWeight = ...
        min(max(depthTaskWeight,0),1);
else
    statusDepthTaskWeight = 0;
end

if isfinite(schedulerMode)
    statusSchedulerMode = schedulerMode;
else
    statusSchedulerMode = 0;
end

statusSafetyValid = double( ...
    isfinite(safetyValid) && ...
    safetyValid > 0.5);

statusControllerEnableSafe = double( ...
    isfinite(controllerEnableSafe) && ...
    controllerEnableSafe > 0.5);

%% 固定顺序状态数组
controllerStatus = [
    statusInputDataValid
    statusCameraModelValid
    statusFocalLengthFresh
    statusKinematicsValid
    statusValidLeft
    statusValidRight
    statusValidStereoQualified
    statusEkfPredictionValid
    statusEkfMeasurementUpdated
    statusDepthTaskWeight
    statusSchedulerMode
    statusSafetyValid
    statusControllerEnableSafe
];

%% 最终机械臂输出许可
armCommandEnable = ...
    all(isfinite(qDot)) && ...
    statusInputDataValid > 0.5 && ...
    statusCameraModelValid > 0.5 && ...
    statusKinematicsValid > 0.5 && ...
    statusValidLeft > 0.5 && ...
    statusSafetyValid > 0.5 && ...
    statusControllerEnableSafe > 0.5;

if armCommandEnable
    jointVelocityCmd = qDot;
end

%% 最终Zoom输出许可
zoomCommandEnable = ...
    all(isfinite(fDotMm)) && ...
    statusInputDataValid > 0.5 && ...
    statusCameraModelValid > 0.5 && ...
    statusFocalLengthFresh > 0.5 && ...
    statusValidLeft > 0.5 && ...
    statusSafetyValid > 0.5 && ...
    statusControllerEnableSafe > 0.5;

if zoomCommandEnable
    focalRateCmdMmPerSec = fDotMm;
end

%% 最终有限值保护
if any(~isfinite(jointVelocityCmd))
    jointVelocityCmd = zeros(7,1);
end

if any(~isfinite(focalRateCmdMmPerSec))
    focalRateCmdMmPerSec = zeros(2,1);
end

if any(~isfinite(controllerStatus))
    controllerStatus = zeros(13,1);
end
end

== matlab function stereo_ibvs_core_backup_20260724_010158/Split Vision Feature ==
  data: visionFeature input; validLeft output; validRight output; pixelMeasurement output; scaleMeasuredRaw output
function [validLeft,validRight,pixelMeasurement,scaleMeasuredRaw] = fcn(visionFeature)
%#codegen
feature = reshape(visionFeature,8,1);
validLeft = feature(1);
validRight = feature(2);
pixelMeasurement = feature(3:6);
scaleMeasuredRaw = feature(7:8);
end

== matlab function stereo_ibvs_core_backup_20260724_010158/Target Velocity Frame Transform ==
  data: vHatW input; vHatCR output; RWCR input
function vHatCR = fcn(vHatW,RWCR)
%#codegen
vHatCR = zeros(3,1);
velocityW = reshape(vHatW,3,1);
rotationCRToW = reshape(RWCR,3,3);
if all(isfinite(velocityW)) && all(isfinite(rotationCRToW(:)))
    vHatCR = rotationCRToW'*velocityW;
end
end

== matlab function stereo_ibvs_core_backup_20260724_010158/02_Camera_and_Zoom_Model/V2_Camera_and_Zoom_Model ==
  data: focalLengthMeasuredMmRaw input; focalLengthMeasuredMm output; focalLengthIsNew input; resetSafe input; cfg_focalLengthHardwareMinMm input; cfg_focalLengthHardwareMaxMm input; cfg_focalLengthWorkingMinMm input; cfg_focalLengthWorkingMaxMm input; cfg_outputPixelPitchXmm input; cfg_outputPixelPitchYmm input; cfg_focalLengthTimeoutFrames input; cfg_numericalEpsilon input; fxMeasuredPx output; fyMeasuredPx output; focalLengthFresh output; focalLengthDataValid output; focalAtWorkingLowerLimit output; focalAtWorkingUpperLimit output; focalAtHardwareLowerLimit output; focalAtHardwareUpperLimit output; focalOutsideWorkingRange output; focalHardwareLimitViolation output; focalRangeUsage output; focalHeadroomMm output; cameraModelValid output
function [ ...
    focalLengthMeasuredMm, ...
    fxMeasuredPx, ...
    fyMeasuredPx, ...
    focalLengthFresh, ...
    focalLengthDataValid, ...
    focalAtWorkingLowerLimit, ...
    focalAtWorkingUpperLimit, ...
    focalAtHardwareLowerLimit, ...
    focalAtHardwareUpperLimit, ...
    focalOutsideWorkingRange, ...
    focalHardwareLimitViolation, ...
    focalRangeUsage, ...
    focalHeadroomMm, ...
    cameraModelValid] = fcn( ...
    focalLengthMeasuredMmRaw, ...
    focalLengthIsNew, ...
    resetSafe, ...
    cfg_focalLengthHardwareMinMm, ...
    cfg_focalLengthHardwareMaxMm, ...
    cfg_focalLengthWorkingMinMm, ...
    cfg_focalLengthWorkingMaxMm, ...
    cfg_outputPixelPitchXmm, ...
    cfg_outputPixelPitchYmm, ...
    cfg_focalLengthTimeoutFrames, ...
    cfg_numericalEpsilon)
%#codegen
% V2 Camera and Zoom Model
%
% 焦距反馈：
% [fL_mm; fR_mm]
%
% 超时后保持最后一次有效焦距，但 focalLengthFresh = false。
% 08模块应在 focalLengthFresh = false 时停止Zoom命令。

%% 固定尺寸输入
focalRaw = reshape(focalLengthMeasuredMmRaw,2,1);

hardwareMin = reshape( ...
    cfg_focalLengthHardwareMinMm,2,1);

hardwareMax = reshape( ...
    cfg_focalLengthHardwareMaxMm,2,1);

workingMin = reshape( ...
    cfg_focalLengthWorkingMinMm,2,1);

workingMax = reshape( ...
    cfg_focalLengthWorkingMaxMm,2,1);

%% 持久状态
persistent lastValidFocalLengthMm
persistent focalLengthReceivedOnce
persistent framesSinceLastValidMessage

if isempty(lastValidFocalLengthMm)
    lastValidFocalLengthMm = zeros(2,1);
    focalLengthReceivedOnce = false;
    framesSinceLastValidMessage = ...
        double(cfg_focalLengthTimeoutFrames);
end

%% 固定尺寸输出
focalLengthMeasuredMm = zeros(2,1);
fxMeasuredPx = zeros(2,1);
fyMeasuredPx = zeros(2,1);

focalLengthFresh = false;
focalLengthDataValid = false;

focalAtWorkingLowerLimit = false(2,1);
focalAtWorkingUpperLimit = false(2,1);
focalAtHardwareLowerLimit = false(2,1);
focalAtHardwareUpperLimit = false(2,1);

focalOutsideWorkingRange = false(2,1);
focalHardwareLimitViolation = false(2,1);

focalRangeUsage = zeros(2,1);
focalHeadroomMm = zeros(2,1);

cameraModelValid = false;

%% 配置检查
numericalConfigurationValid = ...
    isfinite(cfg_numericalEpsilon) && ...
    cfg_numericalEpsilon > 0;

hardwareRangeValid = ...
    all(isfinite(hardwareMin)) && ...
    all(isfinite(hardwareMax)) && ...
    all(hardwareMax > hardwareMin);

workingRangeValid = ...
    all(isfinite(workingMin)) && ...
    all(isfinite(workingMax)) && ...
    all(workingMax > workingMin) && ...
    all(workingMin >= hardwareMin) && ...
    all(workingMax <= hardwareMax);

pixelPitchValid = ...
    isfinite(cfg_outputPixelPitchXmm) && ...
    isfinite(cfg_outputPixelPitchYmm) && ...
    cfg_outputPixelPitchXmm > cfg_numericalEpsilon && ...
    cfg_outputPixelPitchYmm > cfg_numericalEpsilon;

timeoutConfigurationValid = ...
    isfinite(cfg_focalLengthTimeoutFrames) && ...
    cfg_focalLengthTimeoutFrames >= 1;

configurationValid = ...
    numericalConfigurationValid && ...
    hardwareRangeValid && ...
    workingRangeValid && ...
    pixelPitchValid && ...
    timeoutConfigurationValid;

%% 控制输入检查
controlSignalsFinite = ...
    isfinite(focalLengthIsNew) && ...
    isfinite(resetSafe);

%% 复位或更新焦距状态
if ~controlSignalsFinite || resetSafe > 0.5

    lastValidFocalLengthMm = zeros(2,1);
    focalLengthReceivedOnce = false;
    framesSinceLastValidMessage = ...
        double(cfg_focalLengthTimeoutFrames);

else

    rawFinite = all(isfinite(focalRaw));

    rawInsideHardwareRange = ...
        rawFinite && ...
        hardwareRangeValid && ...
        all(focalRaw >= hardwareMin) && ...
        all(focalRaw <= hardwareMax);

    newValidMessage = ...
        focalLengthIsNew > 0.5 && ...
        rawInsideHardwareRange && ...
        configurationValid;

    if newValidMessage

        lastValidFocalLengthMm = focalRaw;
        focalLengthReceivedOnce = true;
        framesSinceLastValidMessage = 0;

    elseif focalLengthReceivedOnce

        maximumCounterValue = ...
            double(cfg_focalLengthTimeoutFrames) + 1;

        framesSinceLastValidMessage = min( ...
            framesSinceLastValidMessage + 1, ...
            maximumCounterValue);
    end
end

%% 输出最近一次有效焦距
if focalLengthReceivedOnce
    focalLengthMeasuredMm = ...
        lastValidFocalLengthMm;
end

%% 焦距新鲜度
focalLengthFresh = ...
    focalLengthReceivedOnce && ...
    framesSinceLastValidMessage < ...
        double(cfg_focalLengthTimeoutFrames);

%% 保存焦距有效性
if focalLengthReceivedOnce && hardwareRangeValid

    focalLengthDataValid = ...
        all(isfinite(focalLengthMeasuredMm)) && ...
        all(focalLengthMeasuredMm >= hardwareMin) && ...
        all(focalLengthMeasuredMm <= hardwareMax);
end

%% 焦距范围状态
if focalLengthReceivedOnce && configurationValid

    focalAtWorkingLowerLimit = ...
        focalLengthMeasuredMm <= workingMin;

    focalAtWorkingUpperLimit = ...
        focalLengthMeasuredMm >= workingMax;

    focalAtHardwareLowerLimit = ...
        focalLengthMeasuredMm <= hardwareMin;

    focalAtHardwareUpperLimit = ...
        focalLengthMeasuredMm >= hardwareMax;

    focalOutsideWorkingRange = ...
        focalLengthMeasuredMm < workingMin | ...
        focalLengthMeasuredMm > workingMax;

    focalHardwareLimitViolation = ...
        focalLengthMeasuredMm < hardwareMin | ...
        focalLengthMeasuredMm > hardwareMax;

    workingRangeWidth = ...
        workingMax - workingMin;

    focalRangeUsage = ...
        (focalLengthMeasuredMm-workingMin) ./ ...
        workingRangeWidth;

    focalRangeUsage = min( ...
        max(focalRangeUsage,zeros(2,1)), ...
        ones(2,1));

    lowerHeadroomMm = ...
        focalLengthMeasuredMm-workingMin;

    upperHeadroomMm = ...
        workingMax-focalLengthMeasuredMm;

    focalHeadroomMm = max( ...
        min(lowerHeadroomMm,upperHeadroomMm), ...
        zeros(2,1));
end

%% 焦距mm转换为像素焦距
cameraModelValid = ...
    configurationValid && ...
    focalLengthDataValid && ...
    ~any(focalHardwareLimitViolation);

if cameraModelValid

    fxMeasuredPx = ...
        focalLengthMeasuredMm ./ ...
        cfg_outputPixelPitchXmm;

    fyMeasuredPx = ...
        focalLengthMeasuredMm ./ ...
        cfg_outputPixelPitchYmm;
end

%% 最终有限值保护
outputFinite = ...
    all(isfinite(focalLengthMeasuredMm)) && ...
    all(isfinite(fxMeasuredPx)) && ...
    all(isfinite(fyMeasuredPx)) && ...
    all(isfinite(focalRangeUsage)) && ...
    all(isfinite(focalHeadroomMm));

if ~outputFinite

    focalLengthMeasuredMm = zeros(2,1);
    fxMeasuredPx = zeros(2,1);
    fyMeasuredPx = zeros(2,1);

    focalLengthFresh = false;
    focalLengthDataValid = false;

    focalAtWorkingLowerLimit = false(2,1);
    focalAtWorkingUpperLimit = false(2,1);
    focalAtHardwareLowerLimit = false(2,1);
    focalAtHardwareUpperLimit = false(2,1);

    focalOutsideWorkingRange = false(2,1);
    focalHardwareLimitViolation = false(2,1);

    focalRangeUsage = zeros(2,1);
    focalHeadroomMm = zeros(2,1);

    cameraModelValid = false;
end
end
